simulink model "model6_no"  (R2022a)
settings: Solver=FixedStepAuto  StartTime=0.0  StopTime=5  FixedStep=1e-5  RelTol=1e-3
model workspace (MAT data in the model file):
  b1 = 10
  b2 = 1500
  downSpringHeight = 10
  g = 9.81
  groundHeight = 100
  k1 = 400
  k2 = 10000000
  m1 = 3.6
  m1IniHeight = 10
  m2 = 3.6
  m3 = 3.6
  upSpringHeight = 10
settings Model: Creator=Tsing  LastModifiedBy=Tsing

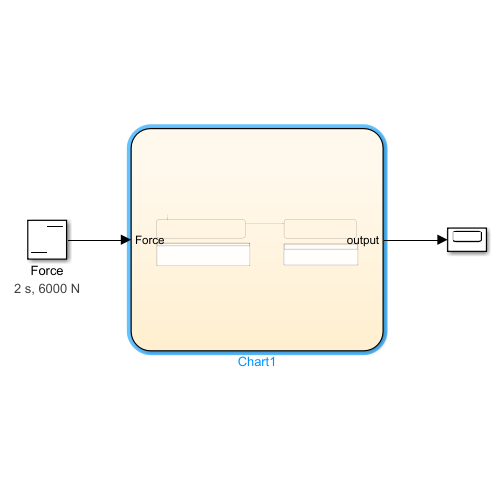
[thumbnail: Simulink's stored preview of the top-level diagram]
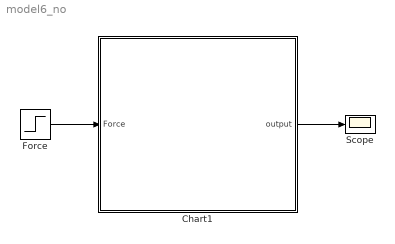
== system model6_no ==
  Chart1 : Stateflow chart  TreatAsAtomicUnit=on
  Force : Step  Time=2  After=6000  SampleTime=0
      settings: AttributesFormatString=%<Time> s, %<After> N
  Scope : Scope
  wires:
  Force/1 -> Chart1/1(Force)
  Chart1/1(output) -> Scope/1

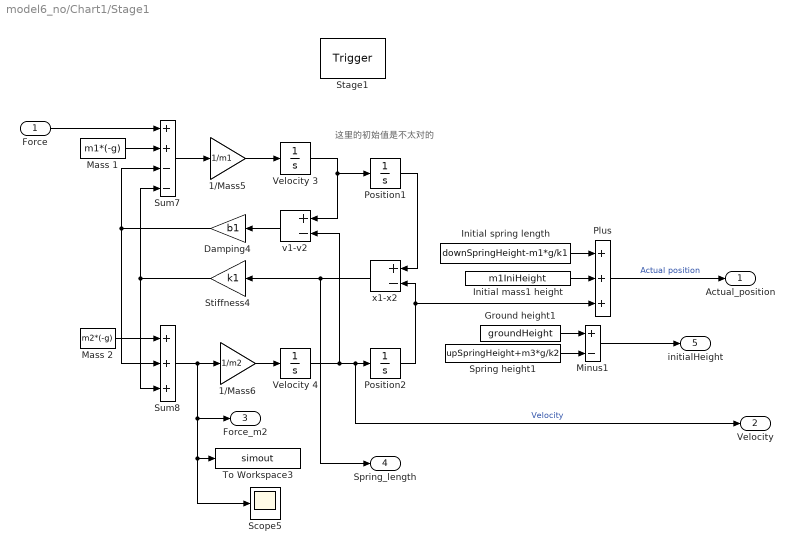
== system model6_no/Chart1/Stage1 ==
  note: 这里的初始值是不太对的
  Force : Inport  OutMin=1  OutMax=1  OutDataTypeStr=double  PortDimensions=1
  Stage1 : TriggerPort  TriggerType=function-call  VariantControl=(inherit)
      settings: CopyFcn=Stateflow.SLINSF.SimulinkMan.removeBlockPreDeleteFcn  PreDeleteFcn=Stateflow.SLINSF.SimulinkMan.unsafePredeleteFcn
  1/Mass5 : Gain  Gain=1/m1  SaturateOnIntegerOverflow=on  OutDataTypeStr=Inherit: Same as input  ParamDataTypeStr=Inherit: Same as input
  1/Mass6 : Gain  Gain=1/m2  SaturateOnIntegerOverflow=on  OutDataTypeStr=Inherit: Same as input  ParamDataTypeStr=Inherit: Same as input
  Damping4 : Gain  Gain=b1  SaturateOnIntegerOverflow=on  OutDataTypeStr=Inherit: Same as input  ParamDataTypeStr=Inherit: Same as input
  Ground height1 : Constant  Value=groundHeight
  Initial mass1 height : Constant  Value=m1IniHeight
  Initial spring length : Constant  Value=downSpringHeight-m1*g/k1
  Mass 1 : Constant  Value=m1*(-g)
  Mass 2 : Constant  Value=m2*(-g)
  Minus1 : Sum  Inputs=+-
  Plus : Sum  Inputs=+++
  Position1 : Integrator
      settings: AttributesFormatString=x0 = %<InitialCondition> m
  Position2 : Integrator
      settings: AttributesFormatString=x0 = %<InitialCondition> m
  Scope5 : Scope
  Spring height1 : Constant  Value=upSpringHeight+m3*g/k2
  Stiffness4 : Gain  Gain=k1  SaturateOnIntegerOverflow=on  OutDataTypeStr=Inherit: Same as input  ParamDataTypeStr=Inherit: Same as input
  Sum7 : Sum  Inputs=++--  InputSameDT=on  SaturateOnIntegerOverflow=on  OutDataTypeStr=Inherit: Same as first input
  Sum8 : Sum  Inputs=+++  InputSameDT=on  SaturateOnIntegerOverflow=on  OutDataTypeStr=Inherit: Same as first input
  To Workspace3 : ToWorkspace  VariableName=simout  SaveFormat=Timeseries  SampleTime=-1
  Velocity 3 : Integrator
      settings: AttributesFormatString=v0 = %<InitialCondition> m/s
  Velocity 4 : Integrator
      settings: AttributesFormatString=v0 = %<InitialCondition> m/s
  v1-v2 : Sum  Inputs=+-
  x1-x2 : Sum  Inputs=+-
  Actual_position : Outport
  Velocity : Outport  Port=2
  Force_m2 : Outport  Port=3
  Spring_length : Outport  Port=4
  initialHeight : Outport  Port=5
  wires:
  Spring height1/1 -> Minus1/2
  Initial mass1 height/1 -> Plus/2
  v1-v2/1 -> Damping4/1
  Sum8/1 -> Force_m2/1, Scope5/1, To Workspace3/1, 1/Mass6/1
  Mass 2/1 -> Sum8/1
  Force/1 -> Sum7/1
  Velocity 3/1 -> Position1/1, v1-v2/1
  1/Mass6/1 -> Velocity 4/1
  Velocity 4/1 -> Velocity/1, Position2/1, v1-v2/2  "Velocity"
  Initial spring length/1 -> Plus/1
  Position1/1 -> x1-x2/1
  Position2/1 -> Plus/3, x1-x2/2
  x1-x2/1 -> Spring_length/1, Stiffness4/1
  Mass 1/1 -> Sum7/2
  1/Mass5/1 -> Velocity 3/1
  Ground height1/1 -> Minus1/1
  Plus/1 -> Actual_position/1  "Actual position"
  Stiffness4/1 -> Sum7/4, Sum8/3
  Sum7/1 -> 1/Mass5/1
  Damping4/1 -> Sum7/3, Sum8/2
  Minus1/1 -> initialHeight/1

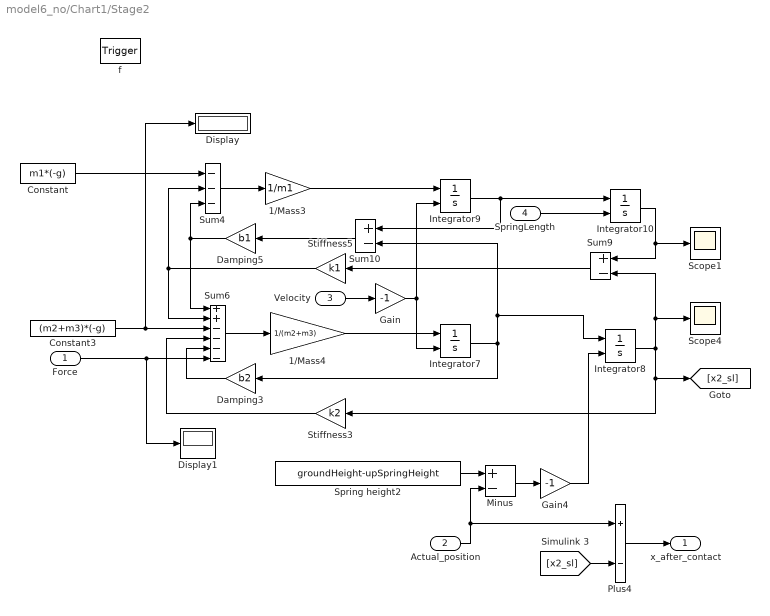
== system model6_no/Chart1/Stage2 ==
  Force : Inport  OutMin=1  OutMax=1  OutDataTypeStr=double  PortDimensions=1
  Actual_position : Inport  Port=2  OutMin=1  OutMax=1  OutDataTypeStr=double  PortDimensions=1
  Velocity : Inport  Port=3  OutMin=1  OutMax=1  OutDataTypeStr=double  PortDimensions=1
  SpringLength : Inport  Port=4  OutMin=1  OutMax=1  OutDataTypeStr=double  PortDimensions=1
  f : TriggerPort  TriggerType=function-call  VariantControl=(inherit)
      settings: CopyFcn=Stateflow.SLINSF.SimulinkMan.removeBlockPreDeleteFcn  PreDeleteFcn=Stateflow.SLINSF.SimulinkMan.unsafePredeleteFcn
  1/Mass3 : Gain  Gain=1/m1  SaturateOnIntegerOverflow=on  OutDataTypeStr=Inherit: Same as input  ParamDataTypeStr=Inherit: Same as input
  1/Mass4 : Gain  Gain=1/(m2+m3)  SaturateOnIntegerOverflow=on  OutDataTypeStr=Inherit: Same as input  ParamDataTypeStr=Inherit: Same as input
  Constant : Constant  Value=m1*(-g)  SampleTime=-1
  Constant3 : Constant  Value=(m2+m3)*(-g)  SampleTime=-1
  Damping3 : Gain  Gain=b2  SaturateOnIntegerOverflow=on  OutDataTypeStr=Inherit: Same as input  ParamDataTypeStr=Inherit: Same as input
  Damping5 : Gain  Gain=b1  SaturateOnIntegerOverflow=on  OutDataTypeStr=Inherit: Same as input  ParamDataTypeStr=Inherit: Same as input
  Display : Display
  Display1 : Display
  Gain : Gain  Gain=-1
  Gain4 : Gain  Gain=-1
  Integrator{7..10} (4 alike) : Integrator  InitialConditionSource=external
      Integrator7 settings: AttributesFormatString=v0 = %<InitialCondition> m/s
      Integrator8 settings: AttributesFormatString=x0 = %<InitialCondition> m
      Integrator9 settings: AttributesFormatString=v0 = %<InitialCondition> m/s
  Minus : Sum  Inputs=+-
  Plus4 : Sum  Inputs=+-
  Scope1 : Scope
  Scope4 : Scope
  Spring height2 : Constant  Value=groundHeight-upSpringHeight  SampleTime=-1
  Stiffness3 : Gain  Gain=k2  SaturateOnIntegerOverflow=on  OutDataTypeStr=Inherit: Same as input  ParamDataTypeStr=Inherit: Same as input
  Stiffness5 : Gain  Gain=k1  SaturateOnIntegerOverflow=on  OutDataTypeStr=Inherit: Same as input  ParamDataTypeStr=Inherit: Same as input
  Sum10 : Sum  Inputs=+-  InputSameDT=on  SaturateOnIntegerOverflow=on  OutDataTypeStr=Inherit: Same as first input
  Sum4 : Sum  Inputs=---  InputSameDT=on  SaturateOnIntegerOverflow=on  OutDataTypeStr=Inherit: Same as first input
  Sum6 : Sum  Inputs=++----  InputSameDT=on  SaturateOnIntegerOverflow=on  OutDataTypeStr=Inherit: Same as first input
  Sum9 : Sum  Inputs=+-  InputSameDT=on  SaturateOnIntegerOverflow=on  OutDataTypeStr=Inherit: Same as first input
  x_after_contact : Outport
  wires:
  Constant/1 -> Sum4/1
  Integrator8/1 -> Scope4/1, Sum9/2, Stiffness3/1, [x2_sl]
  Damping3/1 -> Sum6/5
  Gain4/1 -> Integrator8/2
  Sum4/1 -> 1/Mass3/1
  Sum6/1 -> 1/Mass4/1
  Gain/1 -> Integrator9/2, Integrator7/2
  Plus4/1 -> x_after_contact/1
  Actual_position/1 -> Minus/2, Plus4/1
  Sum9/1 -> Stiffness5/1
  Stiffness5/1 -> Sum6/2, Sum4/2
  1/Mass4/1 -> Integrator7/1
  Integrator7/1 -> Damping3/1, Sum10/2, Integrator8/1
  [x2_sl] -> Plus4/2
  Stiffness3/1 -> Sum6/4
  Damping5/1 -> Sum4/3, Sum6/1
  Force/1 -> Display1/1, Sum6/6
  Constant3/1 -> Display/1, Sum6/3
  Velocity/1 -> Gain/1
  Sum10/1 -> Damping5/1
  Integrator9/1 -> Integrator10/1, Sum10/1
  Integrator10/1 -> Sum9/1, Scope1/1
  1/Mass3/1 -> Integrator9/1
  Minus/1 -> Gain4/1
  Spring height2/1 -> Minus/1
  SpringLength/1 -> Integrator10/2

== stateflow chart model6_no/Chart1 ==
  state BeginStage2
    x_after_contact = Stage2(Force_m2,Actual_position,Velocity,Spring_length);
    output = x_after_contact;
  state Movement
    [Actual_position,Velocity,Force_m2,Spring_length,initialHeight] = Stage1(Force);
    output = Actual_position;
  state [Actual_position,Velocity,Force_m2,Spring_length,initialHeight] = Stage1(Force) [function]
  state x_after_contact = Stage2(Force,Actual_position,Velocity,SpringLength) [function]
  (default) -> Movement
  Movement -> BeginStage2 : [Actual_position >= initialHeight ]
  data: Force function_input double size=1; Actual_position function_output; Velocity function_output; Force_m2 function_output; Spring_length function_output; initialHeight function_output; Force function_input double size=1; Actual_position function_input double size=1; Velocity function_input double size=1; SpringLength function_input double size=1; x_after_contact function_output; Force input; output output; x_after_contact local; Actual_position local; initialHeight local; Force_m2 local; Spring_length local; Velocity local
